simulink model "DMM"  (Simulink 7.3)
settings: Solver=FixedStepDiscrete  SolverMode=SingleTasking  StartTime=0.0  StopTime=49500  RelTol=1e-3
PreLoadFcn:
  | load('MSFTData.mat')
libraries: dspsrcs4 x2
settings Model: Creator=kassama  LastModifiedBy=kassama
settings DataIOCC: SaveOutput=off  SignalLogging=off  SaveTime=off
settings OptimizationCC: InitFltsAndDblsToZero=on
settings DebuggingCC: AlgebraicLoopMsg=error  SingleTaskRateTransMsg=error

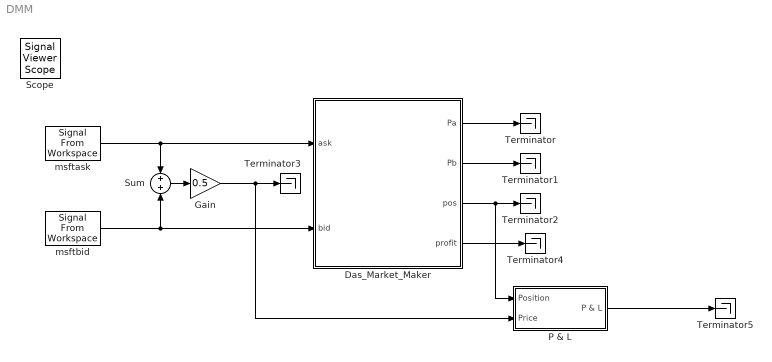
== system DMM ==
  Das_Market_Maker : Stateflow chart
  Gain : Gain  Gain=0.5  ParameterDataType=sfix(16)  ParameterScaling=2^0  OutDataType=sfix(16)  OutScaling=2^0
  P & L : Subsystem
  Sum : Sum  OutDataType=sfix(16)  OutScaling=2^0
  Terminator{,1..5} (6 alike) : Terminator
  msftask : dspsrcs4/Signal From Workspace  SystemSampleTime=-1  X=msftask  Ts=1  nsamps=1  OutputAfterFinalValue=Setting to zero  ignoreOrWarnInputAndFrameLengths=off
  msftbid : dspsrcs4/Signal From Workspace  SystemSampleTime=-1  X=msftbid  Ts=1  nsamps=1  OutputAfterFinalValue=Setting to zero  ignoreOrWarnInputAndFrameLengths=off
  Scope : SignalViewerScope  IOType=viewer  NumInputPorts=3  LegendLocations=|  RefreshTime=0.035000
      | 820.3333      557.6667            89      51.66667
      | 834.3333           390            75      20.33333
      | 771.3333           190           138      20.33333
      settings: ShowLegends=on  YMin=28.275~-6~-0.5  YMax=28.575~5~0.1
  wires:
  msftask/1 -> Das_Market_Maker/1(ask), Sum/1
  msftbid/1 -> Das_Market_Maker/2(bid), Sum/2
  Das_Market_Maker/1(Pa) -> Terminator/1
  Das_Market_Maker/2(Pb) -> Terminator1/1
  Das_Market_Maker/3(pos) -> Terminator2/1, P & L/1(Position)
  Sum/1 -> Gain/1
  Gain/1 -> Terminator3/1, P & L/2(Price)
  Das_Market_Maker/4(profit) -> Terminator4/1
  P & L/1(P & L) -> Terminator5/1

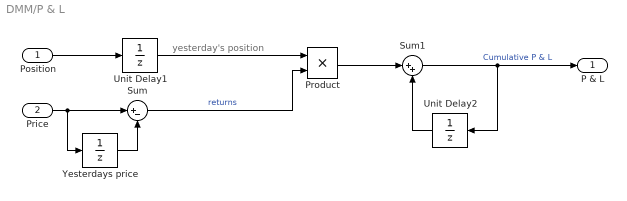
== system DMM/P & L ==
  note: yesterday's position
  Position : Inport  OutDataType=sfix(16)  OutScaling=2^0
  Price : Inport  Port=2  OutDataType=sfix(16)  OutScaling=2^0
  Product : Product  OutDataType=sfix(16)  OutScaling=2^0  RndMeth=Zero
  Sum : Sum  Inputs=|+-  OutDataType=sfix(16)  OutScaling=2^0
  Sum1 : Sum  Inputs=|++  OutDataType=sfix(16)  OutScaling=2^0
  Unit Delay1 : UnitDelay  SampleTime=-1
  Unit Delay2 : UnitDelay  SampleTime=-1
  Yesterdays price : UnitDelay  SampleTime=-1
  P & L : Outport  OutDataType=sfix(16)  OutScaling=2^0
  wires:
  Sum1/1 -> Unit Delay2/1, P & L/1  "Cumulative P & L"
  Unit Delay2/1 -> Sum1/2
  Yesterdays price/1 -> Sum/2
  Product/1 -> Sum1/1
  Unit Delay1/1 -> Product/1
  Sum/1 -> Product/2  "returns"
  Price/1 -> Yesterdays price/1, Sum/1
  Position/1 -> Unit Delay1/1

== stateflow chart Das_Market_Maker ==
  state Quote
  Quote -> (junction 8) [order 1] : % Market sell order
      | [ask<=Pb]
      | {pos+=1;
      | profit-=ask;
      | Prob(Pb,-1);}
  Quote -> (junction 8) [order 2] : % Market buy order
      | [bid >= Pa]
      | {pos-=1;
      | profit+=bid;
      | Prob(Pa,1);}
  (default) -> Quote : {initProb();
      | pos=0;
      | BidAsk();}
  (junction 8) -> (junction 9) : % Recalculate Bid/Ask prices
      | {BidAsk();}
  (junction 9) -> Quote : % Inventory control
      | {icontrol();}
  data: Price function_input double; trade function_input double; ask input double; bid input double; Pa output double; Pb output double; pos output double; V local double size=[111 1]; P local double size=[111 1]; alpha constant double =0.90; profit output double =0; sigma constant double =0.125
  function BidAsk:
    | function BidAsk()
    | 
    | N=111; 
    | % calculate expected value
    | Eorig = sum(V.*P);
    | % round to nearest cent
    | E = round(Eorig*100)/100;
    | t=0.5+0.5*alpha;
    | % find where E occurs in V
    | %[m,EN]=min(abs(V-E));
    | biderror=zeros(N,1);
    | PB=zeros(N,1);
    | % loop over all values of V from Vmin to E
    | for i=1:N
    |     [PB(i), biderror(i)]=bidCalc(i,V,P,t);
    | end
    | 
    | [minerr,ind]=min(biderror);
    | Pb=min(V(ind),E);
    | 
    | askerror=zeros(N,1);
    | PA=zeros(N,1);
    | % loop over all values of V from E to Vmax
    | for i=1:N
    |     [PA(i), askerror(i)]=askCalc(i,V,P,t);
    | end
    | [minerr,ind]=min(askerror);
    | Pa=max(V(ind), E);
    | 
    | %%% ============================== %%%%
    | function [PB,BidErr]=bidCalc(count,V,P,t)
    | N=length(V);
    | a=0;b=0;
    | for i=1:count
    |     a = a+V(i)*P(i);
    | end
    | 
    | for i=count+1:N
    |     b = b+V(i)*P(i);
    | end
    | PB=2*(t*a + (1-t)*b);
    | BidErr = abs(V(count) - PB);
    | 
    | %%%% ============================ %%%%
    | function [PB,BidErr]=askCalc(count,V,P,t)
    | N=length(V);
    | a=0;b=0;
    | for i=1:count-1
    |     a = a+V(i)*P(i);
    | end
    | 
    | for i=count:N
    |     b = b+V(i)*P(i);
    | end
    | PB=2*((1-t)*a + t*b);
    | BidErr = abs(V(count) - PB);
  function Prob(Price,trade):
    | function Prob(Price,trade)
    | % calculate the probability vector
    | % trade is in [-1 0 1] representing sell, flat, buy orders
    | Pold=P;
    | p=(0.5+0.5*alpha);
    | if trade < 0
    |     % sell order received
    |     for i=1:size(V,1)
    |         if V(i,1) < Price
    |             P(i,1)=Pold(i,1)*p;
    |         else
    |             P(i,1)=Pold(i,1)*(1-p);
    |         end
    |     end
    | else %trade > 0
    |     % buy order received
    |     for i=1:size(V,1)
    |         if V(i) > Price
    |             P(i,1)=Pold(i,1)*p;
    |         else
    |             P(i,1)=Pold(i,1)*(1-p);
    |         end
    |     end
    | end
    | 
    | % normalise
    | P=P/sum(P);
  function icontrol:
    | function icontrol()
    | 
    | % sigmoidal function
    | sig = (10*(1+tanh(-3:0.5:3)));
    | xc= 0:length(sig)-1;
    | 
    | % calculate offset
    | offset = round(sign(pos)*interp1(xc,sig,abs(pos),'linear',max(sig)))/100;
    | %offset=0;
    | if pos>0
    |     Pa=Pa-offset;
    |     Pb=Pb-offset;
    | end
  function initProb:
    | function initProb()
    | % initial grid of prices
    | 
    | x0=28.5850;
    | %x0=27.97;
    | V=(27.9:0.01:29)';
    | % normal distn centered around an initial point
    | distn= (1/(sigma*sqrt(2*pi)))*exp(-(V-x0).^2/(2*sigma^2));
    | distn=distn/sum(distn);
    | P=distn;
